simulink model "pipeline_lead_lag"  (R2023a)
settings: Solver=ode45  StartTime=0.0  StopTime=200  MaxStep=0.5  RelTol=1e-3
settings Model: Creator=Theodora  LastModifiedBy=Theodora

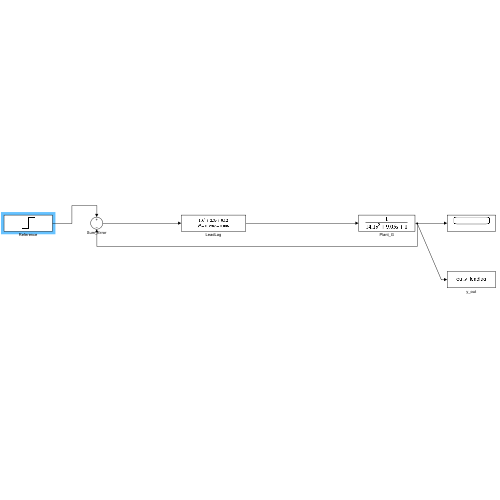
[thumbnail: Simulink's stored preview of the top-level diagram]
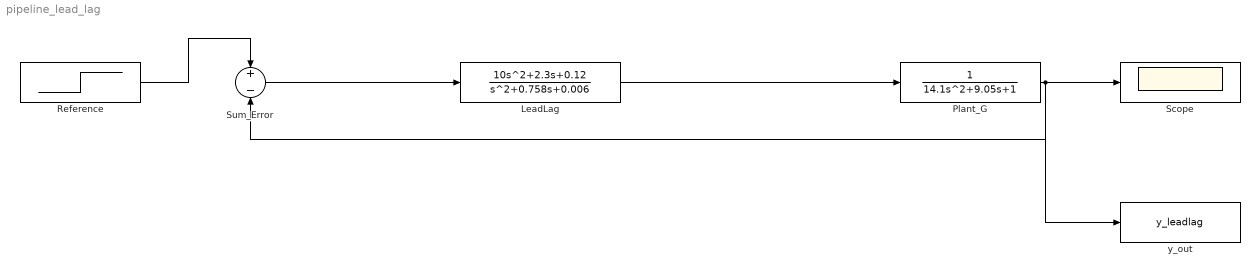
== system pipeline_lead_lag ==
  LeadLag : TransferFcn  Numerator=[10 2.3 0.12]  Denominator=[1 0.758 0.006]
  Plant_G : TransferFcn  Numerator=1  Denominator=[14.1 9.05 1]
  Reference : Step  Time=0  SampleTime=0
  Scope : Scope
  Sum_Error : Sum  Inputs=+-
  y_out : ToWorkspace  VariableName=y_leadlag  SampleTime=-1
  wires:
  Reference/1 -> Sum_Error/1
  Sum_Error/1 -> LeadLag/1
  LeadLag/1 -> Plant_G/1
  Plant_G/1 -> Scope/1, y_out/1, Sum_Error/2
